simulink model "RGB_Color_Component_ManualThresholding"  (R2016a)
settings: Solver=VariableStepAuto  StartTime=0.0  StopTime=10.0  RelTol=1e-3
undefined symbols (not defined in the file): Rec, SDTV
libraries: visionconversions x2, visionsources x2, visionsinks x2
settings Model: Creator=YASARA  LastModifiedBy=YASARA

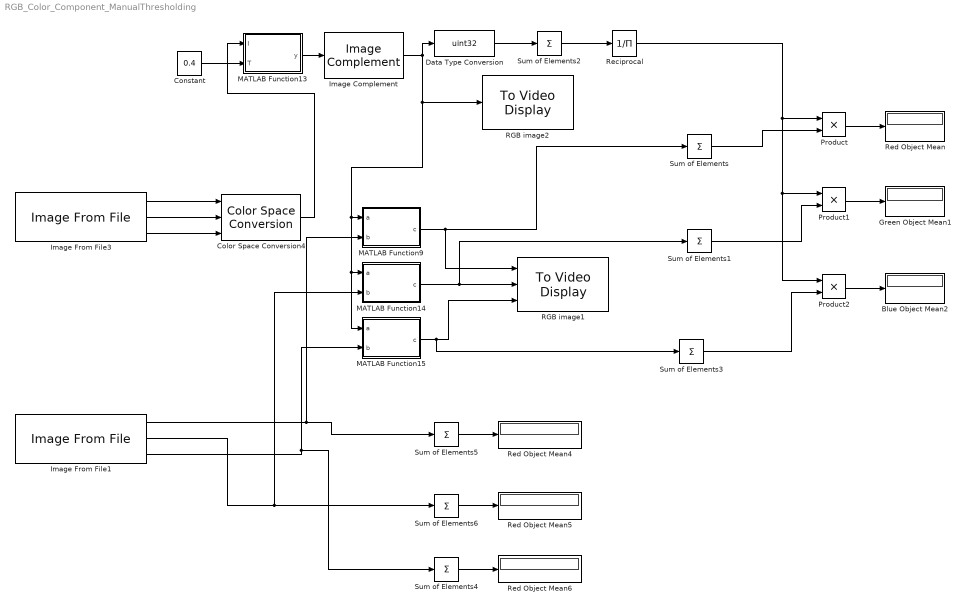
== system RGB_Color_Component_ManualThresholding ==
  Blue Object Mean2 : Display
  Color Space Conversion4 : visionconversions/Color Space  Conversion  conversion=Obsolete  conversionActive=R'G'B' to intensity  wp_str=D65  rec=Rec. 601 (SDTV)  sys=1125/60/2:1  imagePorts=Separate color signals
  Constant : Constant  Value=0.4  SampleTime=1
  Data Type Conversion : DataTypeConversion  OutDataTypeStr=uint32
  Green Object Mean1 : Display
  Image Complement : visionconversions/Image Complement
  Image From File1 : visionsources/Image From File  Tag=vipblks_nd  FileName=C:\Users\YASARA\Desktop\sampl\G200B200R200.jpg  imagePorts=Separate color signals  Ts=1  ImageDataType=Inherit via back propagation  Signed=on  WordLength=16  sdImageDataType=uint(8)  FractionLengthMode=Best precision  FractionLength=15  OutPortLabels=R|G|B
  Image From File3 : visionsources/Image From File  Tag=vipblks_nd  FileName=C:\Users\YASARA\Desktop\sampl\G200B200R200.jpg  imagePorts=Separate color signals  Ts=1  ImageDataType=double  Signed=on  WordLength=16  sdImageDataType=uint(8)  FractionLengthMode=User-defined  FractionLength=15  OutPortLabels=R|G|B
  MATLAB Function13 : MATLAB Function  TreatAsAtomicUnit=on
  MATLAB Function14 : MATLAB Function  TreatAsAtomicUnit=on
  MATLAB Function15 : MATLAB Function  TreatAsAtomicUnit=on
  MATLAB Function9 : MATLAB Function  TreatAsAtomicUnit=on
  Product : Product
  Product1 : Product
  Product2 : Product
  RGB image1 : visionsinks/To Video Display  windowSizeMode=Normal  openAtMdlStart=on  fullScreen=off  videoWindowX=147  videoWindowY=157  saveWindowSize=off  videoWindowWidth=512  videoWindowHeight=384  inputColorFormat=RGB  inputType=Obsolete  imagePorts=Separate color signals  OutputDevice=On-screen video monitor  dataOrg=Column-major  isWindowOpen=off
  RGB image2 : visionsinks/To Video Display  windowSizeMode=Normal  openAtMdlStart=on  fullScreen=off  videoWindowX=147  videoWindowY=157  saveWindowSize=off  videoWindowWidth=512  videoWindowHeight=384  inputColorFormat=RGB  inputType=Obsolete  imagePorts=One multidimensional signal  OutputDevice=On-screen video monitor  dataOrg=Column-major  isWindowOpen=off
  Reciprocal : Product  Inputs=/  OutDataTypeStr=double  RndMeth=Simplest  SaturateOnIntegerOverflow=on
  Red Object Mean{,4..6} (4 alike) : Display
  Sum of Elements{,1..4} (5 alike) : Sum  Inputs=+  AccumDataTypeStr=uint32  OutDataTypeStr=uint32  RndMeth=Nearest
  Sum of Elements5 : Sum  Inputs=+  AccumDataTypeStr=double  OutDataTypeStr=double  RndMeth=Nearest
  Sum of Elements6 : Sum  Inputs=+  AccumDataTypeStr=double  OutDataTypeStr=double  RndMeth=Nearest
  wires:
  MATLAB Function13/1(y) -> Image Complement/1
  Color Space Conversion4/1 -> MATLAB Function13/1(I)
  Sum of Elements/1 -> Product/2
  MATLAB Function9/1(c) -> RGB image1/1, Sum of Elements/1
  MATLAB Function14/1(c) -> RGB image1/2, Sum of Elements1/1
  MATLAB Function15/1(c) -> RGB image1/3, Sum of Elements3/1
  Constant/1 -> MATLAB Function13/2(T)
  Product/1 -> Red Object Mean/1
  Sum of Elements1/1 -> Product1/2
  Product1/1 -> Green Object Mean1/1
  Product2/1 -> Blue Object Mean2/1
  Image Complement/1 -> RGB image2/1, MATLAB Function15/1(a), MATLAB Function14/1(a), MATLAB Function9/1(a), Data Type Conversion/1
  Image From File3/1 -> Color Space Conversion4/1
  Image From File3/2 -> Color Space Conversion4/2
  Image From File3/3 -> Color Space Conversion4/3
  Data Type Conversion/1 -> Sum of Elements2/1
  Sum of Elements3/1 -> Product2/2
  Reciprocal/1 -> Product/1, Product1/1, Product2/1
  Sum of Elements5/1 -> Red Object Mean4/1
  Sum of Elements4/1 -> Red Object Mean6/1
  Sum of Elements6/1 -> Red Object Mean5/1
  Image From File1/2 -> MATLAB Function14/2(b), Sum of Elements6/1
  Image From File1/3 -> MATLAB Function15/2(b), Sum of Elements4/1
  Image From File1/1 -> MATLAB Function9/2(b), Sum of Elements5/1
  Sum of Elements2/1 -> Reciprocal/1

== matlab function RGB_Color_Component_ManualThresholding/MATLAB Function14 ==
  data: a input; b input; c output
function c = fcn(a,b)
%#codegen
c=uint32(a.*b);
return

== matlab function RGB_Color_Component_ManualThresholding/MATLAB Function13 ==
  data: I input; y output; T input
function y = fcn(I,T)
%#codegen
BW = imbinarize(I,double(T));
y = BW;

== matlab function RGB_Color_Component_ManualThresholding/MATLAB Function15 ==
  data: a input; b input; c output
function c = fcn(a,b)
%#codegen
c=uint32(a.*b);
return

== matlab function RGB_Color_Component_ManualThresholding/MATLAB Function9 ==
  data: a input; b input; c output
function c = fcn(a,b)
%#codegen
c=uint32(a.*b);
return
